simulink model "motor_model"  (Simulink 7.3)
settings: Solver=ode45  StartTime=0.0  StopTime=10.0  RelTol=1e-3
values from neighbouring files (symbols this model uses):
  L = 0.032    [az_true.m]
  R = 0.32    [az_true.m]
undefined symbols (not defined in the file or in its folder): n
settings Model: Creator=Sainquake Notebook  LastModifiedBy=Sainquake Notebook

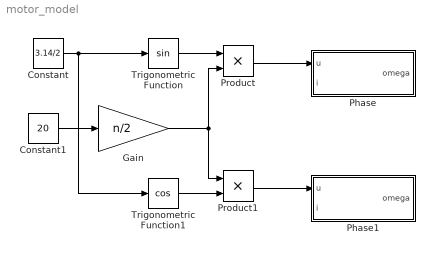
== system motor_model ==
  Constant : Constant  Value=3.14/2  OutDataType=fixdt(1, 16)  OutScaling=2^0
  Constant1 : Constant  Value=20  OutDataType=fixdt(1, 16)  OutScaling=2^0
  Gain : Gain  Gain=n/2  ParameterDataType=fixdt(1, 16)  ParameterScaling=2^0  OutDataType=fixdt(1, 16)  OutScaling=2^0
  Phase : Subsystem
  Phase1 : Subsystem
  Product : Product  OutDataType=fixdt(1, 16)  OutScaling=2^0  RndMeth=Zero
  Product1 : Product  OutDataType=fixdt(1, 16)  OutScaling=2^0  RndMeth=Zero
  Trigonometric Function : Trigonometry
  Trigonometric Function1 : Trigonometry  Operator=cos
  wires:
  Trigonometric Function/1 -> Product/1
  Constant/1 -> Trigonometric Function/1, Trigonometric Function1/1
  Trigonometric Function1/1 -> Product1/2
  Product/1 -> Phase/1(u)
  Product1/1 -> Phase1/1(u)
  Gain/1 -> Product/2, Product1/1
  Constant1/1 -> Gain/1

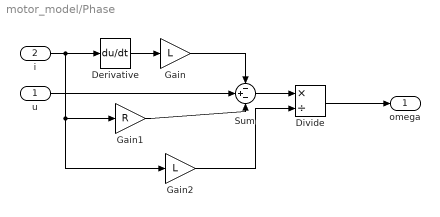
== system motor_model/Phase ==
  u : Inport  OutDataType=fixdt(1, 16)  OutScaling=2^0
  i : Inport  Port=2  OutDataType=fixdt(1, 16)  OutScaling=2^0
  Derivative : Derivative
  Divide : Product  Inputs=*/  OutDataType=fixdt(1, 16)  OutScaling=2^-10
  Gain : Gain  Gain=L  ParameterDataType=fixdt(1, 16)  ParameterScaling=2^0  OutDataType=fixdt(1, 16)  OutScaling=2^0
  Gain1 : Gain  Gain=R  ParameterDataType=fixdt(1, 16)  ParameterScaling=2^0  OutDataType=fixdt(1, 16)  OutScaling=2^0
  Gain2 : Gain  Gain=L  ParameterDataType=fixdt(1, 16)  ParameterScaling=2^0  OutDataType=fixdt(1, 16)  OutScaling=2^0
  Sum : Sum  Inputs=-+-  OutDataType=fixdt(1, 16)  OutScaling=2^0
  omega : Outport  OutDataType=fixdt(1, 16)  OutScaling=2^0
  wires:
  i/1 -> Derivative/1, Gain1/1, Gain2/1
  Derivative/1 -> Gain/1
  u/1 -> Sum/2
  Gain/1 -> Sum/1
  Gain1/1 -> Sum/3
  Sum/1 -> Divide/1
  Gain2/1 -> Divide/2
  Divide/1 -> omega/1

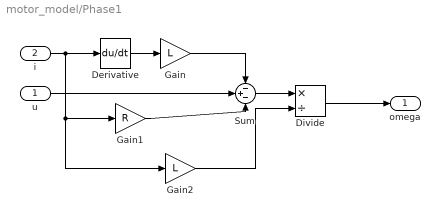
== system motor_model/Phase1 ==
  u : Inport  OutDataType=fixdt(1, 16)  OutScaling=2^0
  i : Inport  Port=2  OutDataType=fixdt(1, 16)  OutScaling=2^0
  Derivative : Derivative
  Divide : Product  Inputs=*/  OutDataType=fixdt(1, 16)  OutScaling=2^-10
  Gain : Gain  Gain=L  ParameterDataType=fixdt(1, 16)  ParameterScaling=2^0  OutDataType=fixdt(1, 16)  OutScaling=2^0
  Gain1 : Gain  Gain=R  ParameterDataType=fixdt(1, 16)  ParameterScaling=2^0  OutDataType=fixdt(1, 16)  OutScaling=2^0
  Gain2 : Gain  Gain=L  ParameterDataType=fixdt(1, 16)  ParameterScaling=2^0  OutDataType=fixdt(1, 16)  OutScaling=2^0
  Sum : Sum  Inputs=-+-  OutDataType=fixdt(1, 16)  OutScaling=2^0
  omega : Outport  OutDataType=fixdt(1, 16)  OutScaling=2^0
  wires:
  Divide/1 -> omega/1
  Gain2/1 -> Divide/2
  Sum/1 -> Divide/1
  Gain1/1 -> Sum/3
  Gain/1 -> Sum/1
  u/1 -> Sum/2
  Derivative/1 -> Gain/1
  i/1 -> Gain2/1, Gain1/1, Derivative/1
